simulink model "model"  (R2015a)
settings: Solver=ode45  StartTime=0.0  StopTime=10.0  RelTol=1e-3
libraries: simulink x1, powerlib x1
settings Model: Creator=Speed Store  LastModifiedBy=Speed Store

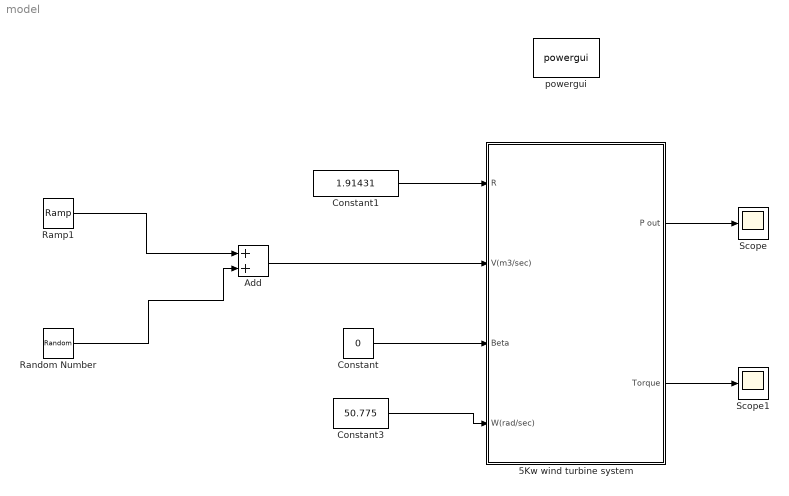
== system model ==
  5Kw wind turbine system : Subsystem  TreatAsAtomicUnit=on
      settings: RTWFcnNameOpts=Use subsystem name  RTWFileNameOpts=Use function name
  Add : Sum
  Constant : Constant  Value=0
  Constant1 : Constant  Value=1.91431
  Constant3 : Constant  Value=50.775
  Ramp1 : simulink/Sources/Ramp  slope=1  start=0  X0=8
  Random Number : RandomNumber  Variance=0.01  SampleTime=0.1
  Scope : Scope
  Scope1 : Scope
  powergui : powerlib/powergui  Priority=1  SimulationMode=Continuous  SolverType=Tustin/Backward Euler (TBE)  SampleTime=50e-6  frequency=60  SPID=off  DisableSnubberDevices=off  DisableRonSwitches=off  DisableVfSwitches=off  SwTol=0  DisplayEquations=off  Interpol=off  methode=off  Ts=100  FunctionMessages=off  echomessages=off  HookPort=off  EnableUseOfTLC=off  x0status=blocks  frequencyindice=60  Pbase=100e6  ErrMax=1e-4  Iterations=50  UnitsV=kV  UnitsW=MW  buscounter=0  RestoreLinks=warning  ResistiveCurrentMeasurement=off  Frange=[0:2:500]  Ylog=off  Xlog=on  ShowGrid=off  save=off  variable=ZData  structure=0  ZoomFFT=off  StartTime=0.0  cycles=1  DisplayStyle=1  fundamental=60  FreqAxis=off  MaxFrequency=1000  frequencyindicesteady=1  RmsSteady=1  display=off
  wires:
  Constant/1 -> 5Kw wind turbine system/3(Beta)
  Constant1/1 -> 5Kw wind turbine system/1(R)
  Constant3/1 -> 5Kw wind turbine system/4(W(rad/sec))
  5Kw wind turbine system/1(P out) -> Scope/1
  5Kw wind turbine system/2(Torque) -> Scope1/1
  Ramp1/1 -> Add/1
  Add/1 -> 5Kw wind turbine system/2(V(m3/sec))
  Random Number/1 -> Add/2

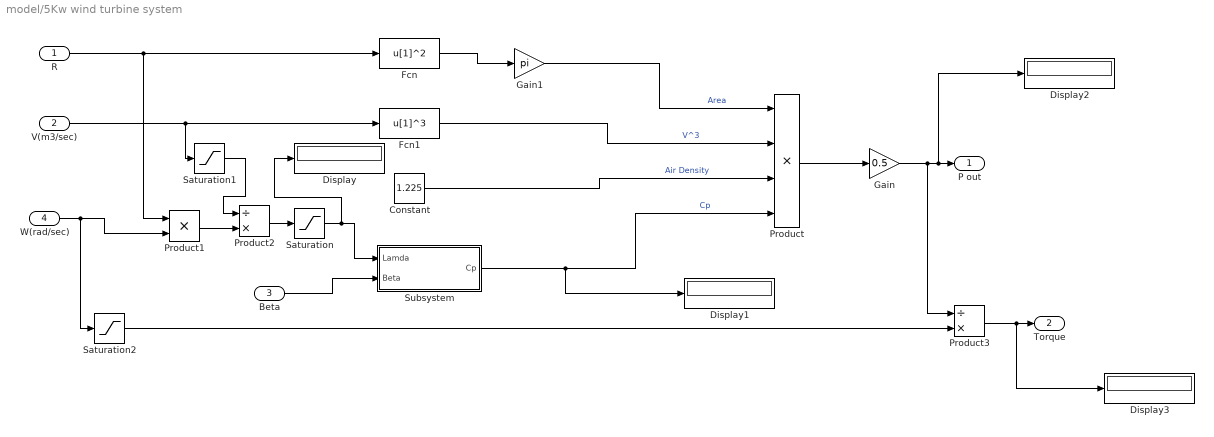
== system model/5Kw wind turbine system ==
  R : Inport
  V(m3/sec) : Inport  Port=2
  Beta : Inport  Port=3
  W(rad/sec) : Inport  Port=4
  Constant : Constant  Value=1.225
  Display{,1..3} (4 alike) : Display
  Fcn : Fcn  Expr=u[1]^2
  Fcn1 : Fcn  Expr=u[1]^3
  Gain : Gain  Gain=0.5
  Gain1 : Gain  Gain=pi
  Product : Product  Inputs=4
  Product1 : Product
  Product2 : Product  Inputs=/*
  Product3 : Product  Inputs=/*
  Saturation : Saturate  UpperLimit=inf  LowerLimit=1e-6
  Saturation1 : Saturate  UpperLimit=inf  LowerLimit=1e-6
  Saturation2 : Saturate  UpperLimit=inf  LowerLimit=1e-6
  Subsystem : Subsystem
  P out : Outport
  Torque : Outport  Port=2
  wires:
  Gain1/1 -> Product/1  "Area"
  Fcn1/1 -> Product/2  "V^3"
  Constant/1 -> Product/3  "Air Density"
  Subsystem/1(Cp) -> Display1/1, Product/4  "Cp"
  Fcn/1 -> Gain1/1
  R/1 -> Product1/1, Fcn/1
  Beta/1 -> Subsystem/2(Beta)
  W(rad/sec)/1 -> Saturation2/1, Product1/2
  V(m3/sec)/1 -> Saturation1/1, Fcn1/1
  Product2/1 -> Saturation/1
  Product1/1 -> Product2/2
  Saturation/1 -> Display/1, Subsystem/1(Lamda)
  Saturation1/1 -> Product2/1
  Saturation2/1 -> Product3/2
  Product/1 -> Gain/1
  Gain/1 -> Display2/1, P out/1, Product3/1
  Product3/1 -> Display3/1, Torque/1

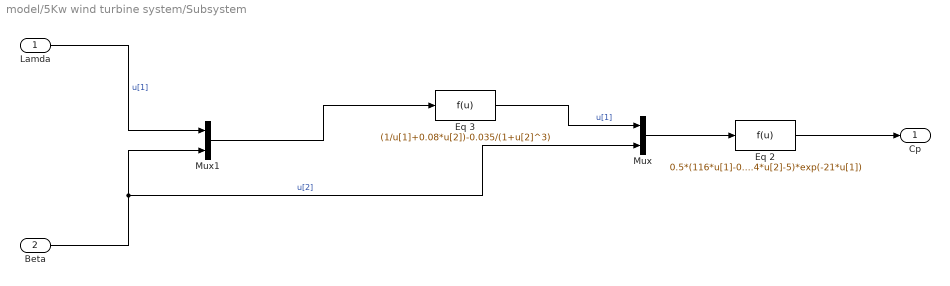
== system model/5Kw wind turbine system/Subsystem ==
  Lamda : Inport
  Beta : Inport  Port=2
  Eq 2 : Fcn  Expr=0.5*(116*u[1]-0.4*u[2]-5)*exp(-21*u[1])
  Eq 3 : Fcn  Expr=(1/u[1]+0.08*u[2])-0.035/(1+u[2]^3)
  Mux : Mux  Inputs=2
  Mux1 : Mux  Inputs=2
  Cp : Outport
  wires:
  Mux/1 -> Eq 2/1
  Eq 2/1 -> Cp/1
  Lamda/1 -> Mux1/1  "u[1]"
  Eq 3/1 -> Mux/1  "u[1]"
  Beta/1 -> Mux/2, Mux1/2  "u[2]"
  Mux1/1 -> Eq 3/1
